simulink model "SimNL"  (R2016b)
settings: Solver=VariableStepAuto  StartTime=0.0  StopTime=10  FixedStep=SampleTime  RelTol=1e-3
undefined symbols (not defined in the file): AC, Sim
libraries: Surf_Lib x7, OpenFlightUtilLib x5, SimCoreLib x2, EnvLib x1
settings Model: Creator=Paul Freeman  LastModifiedBy=rega0051
settings DataIOCC: SaveState=on
settings OptimizationCC: ExpressionDepthLimit=2147483647  LifeSpan=inf
settings DebuggingCC: SignalInfNanChecking=warning  SaveWithParameterizedLinksMsg=none  UnderspecifiedInitializationDetection=Classic  MergeDetectMultiDrivingBlocksExec=none  CheckMatrixSingularityMsg=warning  UnnecessaryDatatypeConvMsg=warning  FcnCallInpInsideContextMsg=warning  UnconnectedInputMsg=none  UnconnectedOutputMsg=none  UnconnectedLineMsg=none  SFcnCompatibilityMsg=warning  UniqueDataStoreMsg=warning  StateNameClashWarn=warning  SFUnexpectedBacktrackingDiag=warning  SFNoUnconditionalDefaultTransitionDiag=warning  SFExecutionAtInitializationDiag=none
settings HardwareCC: ProdBitPerPointer=32  ProdBitPerSizeT=32  ProdBitPerPtrDiffT=32  ProdLargestAtomicFloat=None  ProdWordSize=32  ProdHWDeviceType=Custom Processor->Custom
settings GRTTargetCC: TargetLangStandard=C89/C90 (ANSI)  GeneratePreprocessorConditionals=Disable all  CombineOutputUpdateFcns=off  GRTInterface=on
settings ConfigComp: CovMetricSettings=dw  CovHtmlReporting=on  CovSaveCumulativeToWorkspaceVar=on  CovSaveSingleToWorkspaceVar=on  CovExternalEMLEnable=off  CovSFcnEnable=off

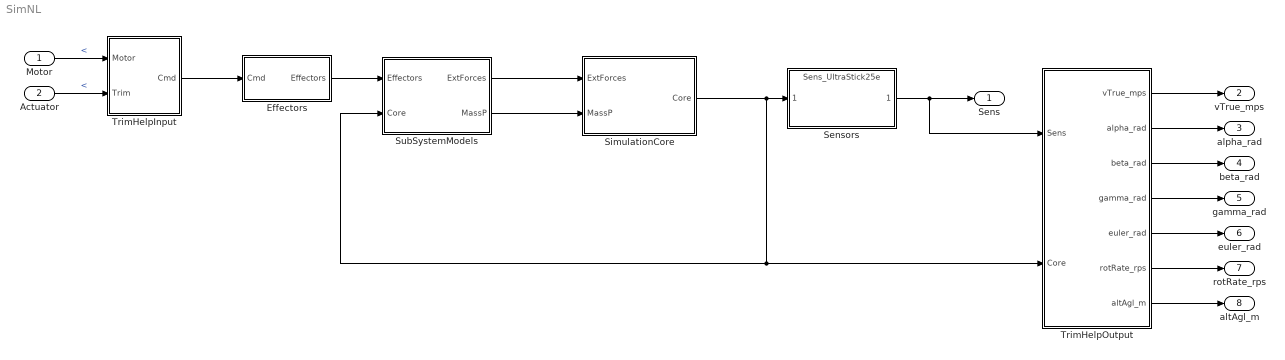
== system SimNL ==
  Motor : Inport
  Actuator : Inport  Port=2
  Effectors : Subsystem  TreatAsAtomicUnit=on
  Sensors : ModelReference  ModelNameDialog=Sens_UltraStick25e.slx  SimulationMode=Normal  ModelReferenceVersion=1.71
  SimulationCore : Subsystem
  SubSystemModels : Subsystem
  TrimHelpInput : Subsystem
  TrimHelpOutput : Subsystem
  Sens : Outport  OutDataTypeStr=Bus: BusSens
  vTrue_mps : Outport  Port=2
  alpha_rad : Outport  Port=3
  beta_rad : Outport  Port=4
  gamma_rad : Outport  Port=5
  euler_rad : Outport  Port=6
  rotRate_rps : Outport  Port=7
  altAgl_m : Outport  Port=8
  wires:
  SimulationCore/1(Core) -> TrimHelpOutput/2(Core), SubSystemModels/2(Core), Sensors/1
  Actuator/1 -> TrimHelpInput/2(Trim)  "<"
  Motor/1 -> TrimHelpInput/1(Motor)  "<"
  TrimHelpInput/1(Cmd) -> Effectors/1(Cmd)
  SubSystemModels/1(ExtForces) -> SimulationCore/1(ExtForces)
  SubSystemModels/2(MassP) -> SimulationCore/2(MassP)
  Sensors/1 -> TrimHelpOutput/1(Sens), Sens/1
  TrimHelpOutput/1(vTrue_mps) -> vTrue_mps/1
  TrimHelpOutput/2(alpha_rad) -> alpha_rad/1
  TrimHelpOutput/3(beta_rad) -> beta_rad/1
  TrimHelpOutput/4(gamma_rad) -> gamma_rad/1
  TrimHelpOutput/5(euler_rad) -> euler_rad/1
  TrimHelpOutput/6(rotRate_rps) -> rotRate_rps/1
  TrimHelpOutput/7(altAgl_m) -> altAgl_m/1
  Effectors/1(Effectors) -> SubSystemModels/1(Effectors)

== system SimNL/Effectors ==
  Cmd : Inport
  Bus Creator : BusCreator  Inputs=3  OutDataTypeStr=Bus: BusEff
      settings: AttributesFormatString=%<OutDataTypeStr>  InheritFromInputs=off
  ControlSurfaces : Subsystem
  MotorModels : Subsystem
  Effectors : Outport
  wires:
  ControlSurfaces/1(Act) -> Bus Creator/2
  MotorModels/1(Throttle) -> Bus Creator/1
  Cmd/1 -> MotorModels/1(Cmd), ControlSurfaces/1(Cmd)
  ControlSurfaces/2(Surf) -> Bus Creator/3
  Bus Creator/1 -> Effectors/1  "BusEff"

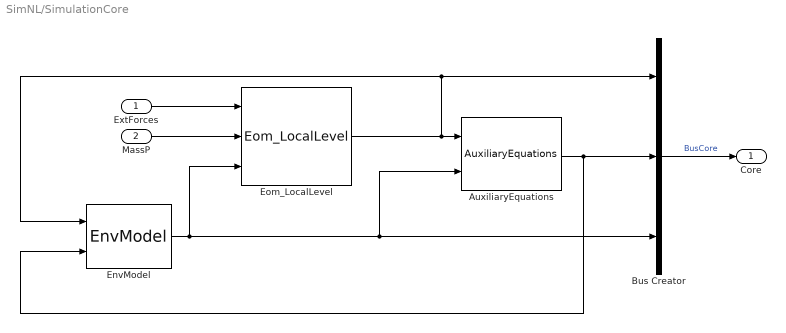
== system SimNL/SimulationCore ==
  ExtForces : Inport
  MassP : Inport  Port=2
  AuxiliaryEquations : SimCoreLib/AuxiliaryEquations
  Bus Creator : BusCreator  Inputs=3  OutDataTypeStr=Bus: BusCore
      settings: AttributesFormatString=%<OutDataTypeStr>
  EnvModel : EnvLib/EnvModel
  Eom_LocalLevel : SimCoreLib/Eom_LocalLevel  SystemSampleTime=-1
  Core : Outport
  wires:
  ExtForces/1 -> Eom_LocalLevel/1
  EnvModel/1 -> AuxiliaryEquations/2, Bus Creator/3, Eom_LocalLevel/3
  Bus Creator/1 -> Core/1  "BusCore"
  MassP/1 -> Eom_LocalLevel/2
  Eom_LocalLevel/1 -> EnvModel/1, Bus Creator/1, AuxiliaryEquations/1
  AuxiliaryEquations/1 -> EnvModel/2, Bus Creator/2

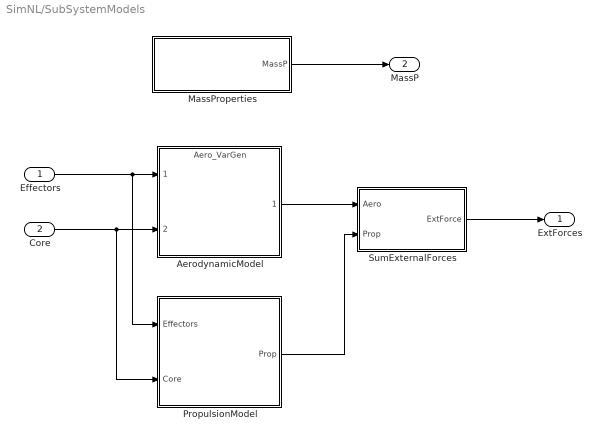
== system SimNL/SubSystemModels ==
  Effectors : Inport
  Core : Inport  Port=2
  AerodynamicModel : ModelReference  ModelNameDialog=Aero_VarGen  SimulationMode=Normal  Variant=on  ModelReferenceVersion=1.70
  MassProperties : Subsystem
  PropulsionModel : Subsystem
  SumExternalForces : Subsystem
  ExtForces : Outport
  MassP : Outport  Port=2
  wires:
  MassProperties/1(MassP) -> MassP/1
  AerodynamicModel/1 -> SumExternalForces/1(Aero)
  SumExternalForces/1(ExtForce) -> ExtForces/1
  PropulsionModel/1(Prop) -> SumExternalForces/2(Prop)
  Effectors/1 -> PropulsionModel/1(Effectors), AerodynamicModel/1
  Core/1 -> PropulsionModel/2(Core), AerodynamicModel/2

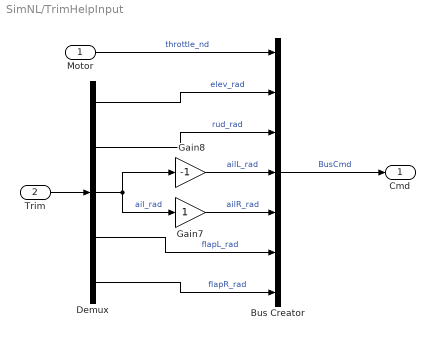
== system SimNL/TrimHelpInput ==
  Motor : Inport
  Trim : Inport  Port=2
  Bus Creator : BusCreator  Inputs=7  OutDataTypeStr=Bus: BusCmd
      settings: AttributesFormatString=%<OutDataTypeStr>
  Demux : Demux  Outputs=5
  Gain7 : Gain
  Gain8 : Gain  Gain=-1
  Cmd : Outport
  wires:
  Motor/1 -> Bus Creator/1  "throttle_nd"
  Demux/2 -> Bus Creator/3  "rud_rad"
  Demux/1 -> Bus Creator/2  "elev_rad"
  Trim/1 -> Demux/1
  Demux/5 -> Bus Creator/7  "flapR_rad"
  Demux/3 -> Gain7/1, Gain8/1  "ail_rad"
  Demux/4 -> Bus Creator/6  "flapL_rad"
  Gain7/1 -> Bus Creator/5  "ailR_rad"
  Gain8/1 -> Bus Creator/4  "ailL_rad"
  Bus Creator/1 -> Cmd/1  "BusCmd"

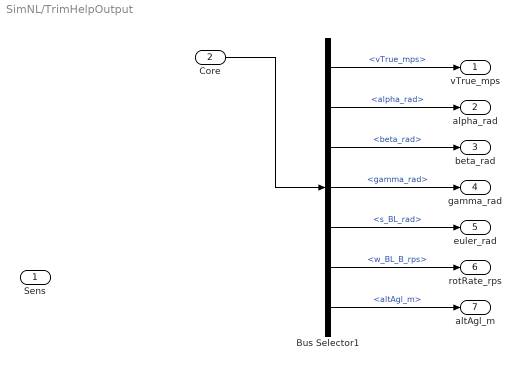
== system SimNL/TrimHelpOutput ==
  Sens : Inport
  Core : Inport  Port=2
  Bus Selector1 : BusSelector  OutputSignals=BusAux.BusFlow.vTrue_mps,BusAux.BusFlow.alpha_rad,BusAux.BusFlow.beta_rad,BusAux.BusNav.gamma_rad,BusEom.s_BL_rad,BusEom.w_BL_B_rps,BusAux.BusNav.altAgl_m
  vTrue_mps : Outport
  alpha_rad : Outport  Port=2
  beta_rad : Outport  Port=3
  gamma_rad : Outport  Port=4
  euler_rad : Outport  Port=5
  rotRate_rps : Outport  Port=6
  altAgl_m : Outport  Port=7
  wires:
  Core/1 -> Bus Selector1/1
  Bus Selector1/1 -> vTrue_mps/1  "<vTrue_mps>"
  Bus Selector1/3 -> beta_rad/1  "<beta_rad>"
  Bus Selector1/2 -> alpha_rad/1  "<alpha_rad>"
  Bus Selector1/4 -> gamma_rad/1  "<gamma_rad>"
  Bus Selector1/5 -> euler_rad/1  "<s_BL_rad>"
  Bus Selector1/6 -> rotRate_rps/1  "<w_BL_B_rps>"
  Bus Selector1/7 -> altAgl_m/1  "<altAgl_m>"

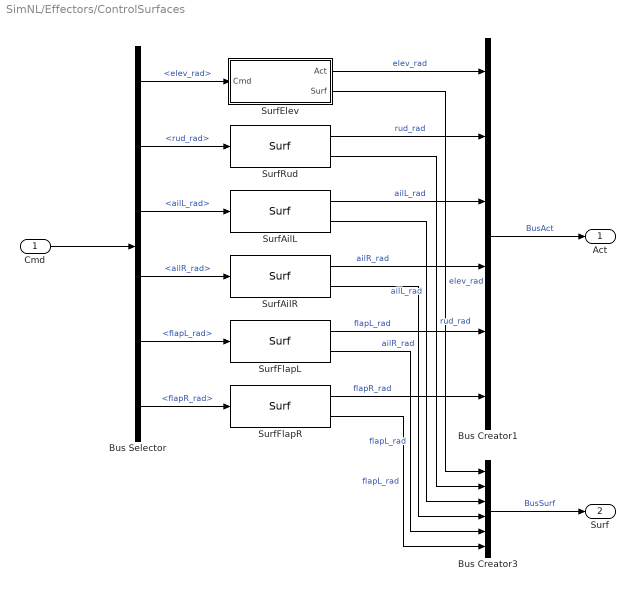
== system SimNL/Effectors/ControlSurfaces ==
  Cmd : Inport
  Bus Creator1 : BusCreator  Inputs=6  OutDataTypeStr=Bus: BusAct
      settings: AttributesFormatString=%<OutDataTypeStr>  InheritFromInputs=off
  Bus Creator3 : BusCreator  Inputs=6  OutDataTypeStr=Bus: BusSurf
      settings: AttributesFormatString=%<OutDataTypeStr>  InheritFromInputs=off
  Bus Selector : BusSelector  OutputSignals=elev_rad,rud_rad,ailL_rad,ailR_rad,flapL_rad,flapR_rad
  SurfAilL : Surf_Lib/Surf  surf=AC.Surf.ailL
  SurfAilR : Surf_Lib/Surf  surf=AC.Surf.ailR
  SurfElev : Subsystem  AncestorBlock=Surf_Lib/Surf  mask{surf=AC.Surf.elev}
      mask prompts: surf "Surface Structure:"
  SurfFlapL : Surf_Lib/Surf  surf=AC.Surf.flapL
  SurfFlapR : Surf_Lib/Surf  surf=AC.Surf.flapR
  SurfRud : Surf_Lib/Surf  surf=AC.Surf.rud
  Act : Outport
  Surf : Outport  Port=2
  wires:
  Bus Creator1/1 -> Act/1  "BusAct"
  Cmd/1 -> Bus Selector/1
  Bus Selector/1 -> SurfElev/1(Cmd)  "<elev_rad>"
  Bus Selector/2 -> SurfRud/1  "<rud_rad>"
  Bus Selector/3 -> SurfAilL/1  "<ailL_rad>"
  SurfAilL/1 -> Bus Creator1/3  "ailL_rad"
  Bus Selector/5 -> SurfFlapL/1  "<flapL_rad>"
  SurfFlapL/1 -> Bus Creator1/5  "flapL_rad"
  SurfAilR/1 -> Bus Creator1/4  "ailR_rad"
  SurfFlapR/1 -> Bus Creator1/6  "flapR_rad"
  Bus Selector/6 -> SurfFlapR/1  "<flapR_rad>"
  SurfRud/1 -> Bus Creator1/2  "rud_rad"
  Bus Selector/4 -> SurfAilR/1  "<ailR_rad>"
  SurfElev/2(Surf) -> Bus Creator3/1  "elev_rad"
  SurfRud/2 -> Bus Creator3/2  "rud_rad"
  SurfAilL/2 -> Bus Creator3/3  "ailL_rad"
  SurfAilR/2 -> Bus Creator3/4  "ailR_rad"
  SurfFlapL/2 -> Bus Creator3/5  "flapL_rad"
  SurfFlapR/2 -> Bus Creator3/6  "flapL_rad"
  Bus Creator3/1 -> Surf/1  "BusSurf"
  SurfElev/1(Act) -> Bus Creator1/1  "elev_rad"

== system SimNL/Effectors/MotorModels ==
  Cmd : Inport  OutDataTypeStr=double
  Bus Creator : BusCreator  Inputs=1
  Bus Selector1 : BusSelector  OutputSignals=throttle_nd
  Throttle : Outport
  wires:
  Cmd/1 -> Bus Selector1/1
  Bus Selector1/1 -> Bus Creator/1  "<throttle_nd>"
  Bus Creator/1 -> Throttle/1  "BusThrot"

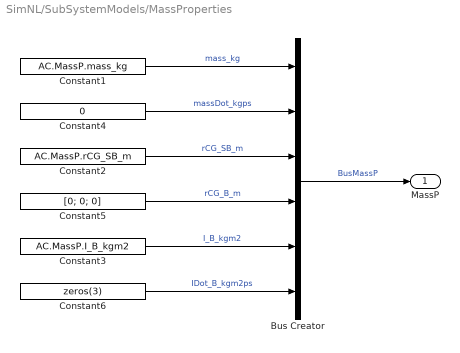
== system SimNL/SubSystemModels/MassProperties ==
  Bus Creator : BusCreator  Inputs=6  OutDataTypeStr=Bus: BusMassP
      settings: AttributesFormatString=%<OutDataTypeStr>
  Constant1 : Constant  Value=AC.MassP.mass_kg
      settings: AttributesFormatString=%<Value>
  Constant2 : Constant  Value=AC.MassP.rCG_SB_m
      settings: AttributesFormatString=%<Value>
  Constant3 : Constant  Value=AC.MassP.I_B_kgm2
      settings: AttributesFormatString=%<Value>
  Constant4 : Constant  Value=0
      settings: AttributesFormatString=%<Value>
  Constant5 : Constant  Value=[0; 0; 0]
      settings: AttributesFormatString=%<Value>
  Constant6 : Constant  Value=zeros(3)
      settings: AttributesFormatString=%<Value>
  MassP : Outport
  wires:
  Bus Creator/1 -> MassP/1  "BusMassP"
  Constant1/1 -> Bus Creator/1  "mass_kg"
  Constant2/1 -> Bus Creator/3  "rCG_SB_m"
  Constant3/1 -> Bus Creator/5  "I_B_kgm2"
  Constant4/1 -> Bus Creator/2  "massDot_kgps"
  Constant5/1 -> Bus Creator/4  "rCG_B_m"
  Constant6/1 -> Bus Creator/6  "IDot_B_kgm2ps"

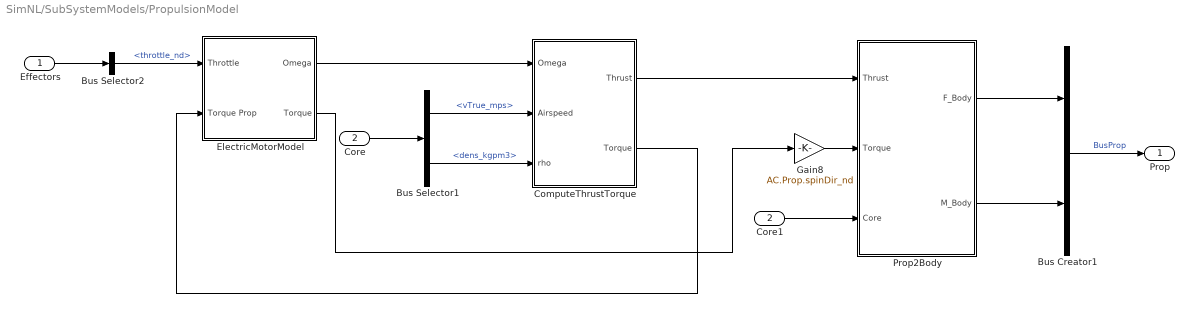
== system SimNL/SubSystemModels/PropulsionModel ==
  Effectors : Inport  OutDataTypeStr=double
  Core : Inport  Port=2
  Bus Selector1 : BusSelector  OutputSignals=BusAux.BusFlow.vTrue_mps,BusEnv.BusAtmos.dens_kgpm3
  Bus Selector2 : BusSelector  OutputSignals=BusThrot.throttle_nd
  Bus Creator1 : BusCreator  Inputs=2  OutDataTypeStr=Bus: BusProp
      settings: AttributesFormatString=%<OutDataTypeStr>
  ComputeThrustTorque : Subsystem
  Core1 : InportShadow  Port=2
  ElectricMotorModel : Subsystem  mask{motor=AC.Motor}
      mask prompts: motor "Motor Parameter Structure:"
  Gain8 : Gain  Gain=AC.Prop.spinDir_nd  SaturateOnIntegerOverflow=on  OutDataTypeStr=Inherit: Same as input  ParamDataTypeStr=Inherit: Same as input
      settings: AttributesFormatString=%<Gain>
  Prop2Body : Subsystem
  Prop : Outport
  wires:
  Core/1 -> Bus Selector1/1
  Prop2Body/2(M_Body) -> Bus Creator1/2
  ComputeThrustTorque/1(Thrust) -> Prop2Body/1(Thrust)
  Bus Selector1/1 -> ComputeThrustTorque/2(Airspeed)  "<vTrue_mps>"
  Prop2Body/1(F_Body) -> Bus Creator1/1
  Core1/1 -> Prop2Body/3(Core)
  Bus Creator1/1 -> Prop/1  "BusProp"
  Bus Selector1/2 -> ComputeThrustTorque/3(rho)  "<dens_kgpm3>"
  ElectricMotorModel/2(Torque) -> Gain8/1
  ComputeThrustTorque/2(Torque) -> ElectricMotorModel/2(Torque Prop)
  Effectors/1 -> Bus Selector2/1
  Gain8/1 -> Prop2Body/2(Torque)
  Bus Selector2/1 -> ElectricMotorModel/1(Throttle)  "<throttle_nd>"
  ElectricMotorModel/1(Omega) -> ComputeThrustTorque/1(Omega)

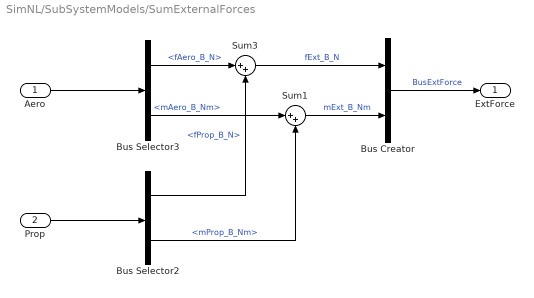
== system SimNL/SubSystemModels/SumExternalForces ==
  Aero : Inport
  Prop : Inport  Port=2
  Bus Selector2 : BusSelector  OutputSignals=fProp_B_N,mProp_B_Nm
  Bus Selector3 : BusSelector  OutputSignals=fAero_B_N,mAero_B_Nm
  Bus Creator : BusCreator  Inputs=2  OutDataTypeStr=Bus: BusExtForce
      settings: AttributesFormatString=%<OutDataTypeStr>
  Sum1 : Sum  Inputs=|++  SaturateOnIntegerOverflow=on
  Sum3 : Sum  Inputs=|++  SaturateOnIntegerOverflow=on
  ExtForce : Outport
  wires:
  Sum1/1 -> Bus Creator/2  "mExt_B_Nm"
  Sum3/1 -> Bus Creator/1  "fExt_B_N"
  Bus Creator/1 -> ExtForce/1  "BusExtForce"
  Prop/1 -> Bus Selector2/1
  Bus Selector2/1 -> Sum3/2  "<fProp_B_N>"
  Bus Selector2/2 -> Sum1/2  "<mProp_B_Nm>"
  Aero/1 -> Bus Selector3/1
  Bus Selector3/1 -> Sum3/1  "<fAero_B_N>"
  Bus Selector3/2 -> Sum1/1  "<mAero_B_Nm>"

== system SimNL/Effectors/ControlSurfaces/SurfElev ==
  Cmd : Inport
  LinkageModel : Subsystem  BlockChoice=LinkageModel_Lin
      settings: AttributesFormatString=%<BlockChoice>  TemplateBlock=Surf_Lib/LinkageModel  MemberBlocks=LinkageModel_Lin,LinkageModel_NL,LinkageModel_Pass
  ServoModel : Subsystem  BlockChoice=ServoModel_2ndLin
      settings: AttributesFormatString=%<BlockChoice>  TemplateBlock=Surf_Lib/ServoModel  MemberBlocks=ServoModel_1stLin,ServoModel_1stNL,ServoModel_2ndLin,ServoModel_2ndNL
  Act : Outport
  Surf : Outport  Port=2
  wires:
  LinkageModel/1(Surf) -> Surf/1
  ServoModel/1(Act) -> Act/1, LinkageModel/1(Act)
  Cmd/1 -> ServoModel/1(Cmd)

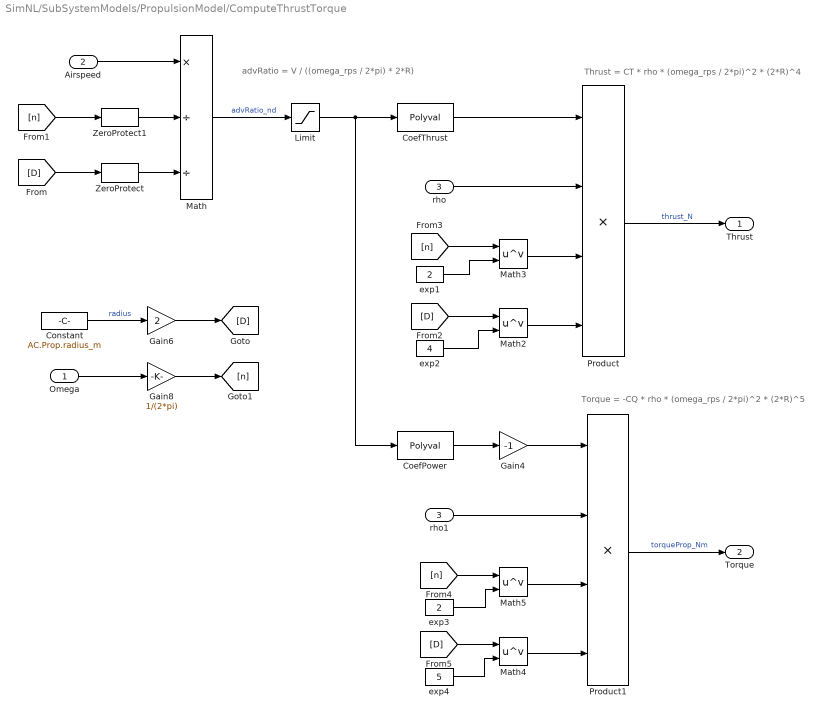
== system SimNL/SubSystemModels/PropulsionModel/ComputeThrustTorque ==
  note: advRatio = V / ((omega_rps / 2*pi) * 2*R)
  note: Thrust = CT * rho * (omega_rps / 2*pi)^2 * (2*R)^4
  note: Torque = -CQ * rho * (omega_rps / 2*pi)^2 * (2*R)^5
  Omega : Inport  OutDataTypeStr=double
  Airspeed : Inport  Port=2  OutDataTypeStr=double
  rho : Inport  Port=3  OutDataTypeStr=double
  CoefPower : Polyval  Coefs=AC.Prop.CQ
      settings: AttributesFormatString=%<Coefs>
  CoefThrust : Polyval  Coefs=AC.Prop.CT
      settings: AttributesFormatString=%<Coefs>
  Constant : Constant  Value=AC.Prop.radius_m
      settings: AttributesFormatString=%<Value>
  Gain4 : Gain  Gain=-1  SaturateOnIntegerOverflow=on  OutDataTypeStr=Inherit: Same as input  ParamDataTypeStr=Inherit: Same as input
  Gain6 : Gain  Gain=2  SaturateOnIntegerOverflow=on  OutDataTypeStr=Inherit: Same as input  ParamDataTypeStr=Inherit: Same as input
  Gain8 : Gain  Gain=1/(2*pi)  SaturateOnIntegerOverflow=on  OutDataTypeStr=Inherit: Same as input  ParamDataTypeStr=Inherit: Same as input
      settings: AttributesFormatString=%<Gain>
  Limit : Saturate  UpperLimit=0.7  LowerLimit=0
  Math : Product  Inputs=*//  SaturateOnIntegerOverflow=on  InputSameDT=on  OutDataTypeStr=Inherit: Same as first input
  Math{2..5} (4 alike) : Math  Operator=pow  SaturateOnIntegerOverflow=on
  Product : Product  Inputs=4  SaturateOnIntegerOverflow=on  InputSameDT=on  OutDataTypeStr=Inherit: Same as first input
  Product1 : Product  Inputs=4  SaturateOnIntegerOverflow=on  InputSameDT=on  OutDataTypeStr=Inherit: Same as first input
  ZeroProtect : OpenFlightUtilLib/Math/ZeroProtect  epsilon=eps
  ZeroProtect1 : OpenFlightUtilLib/Math/ZeroProtect  epsilon=eps
  exp1 : Constant  Value=2
  exp2 : Constant  Value=4
  exp3 : Constant  Value=2
  exp4 : Constant  Value=5
  rho1 : InportShadow  Port=3  OutDataTypeStr=double
  Thrust : Outport
  Torque : Outport  Port=2
  wires:
  CoefPower/1 -> Gain4/1
  CoefThrust/1 -> Product/1
  Product/1 -> Thrust/1  "thrust_N"
  Math2/1 -> Product/4
  exp2/1 -> Math2/2
  Math3/1 -> Product/3
  Math/1 -> Limit/1  "advRatio_nd"
  rho/1 -> Product/2
  Airspeed/1 -> Math/1
  Product1/1 -> Torque/1  "torqueProp_Nm"
  Limit/1 -> CoefThrust/1, CoefPower/1
  [n] -> Math3/1
  [D] -> Math2/1
  exp1/1 -> Math3/2
  Math4/1 -> Product1/4
  exp4/1 -> Math4/2
  Math5/1 -> Product1/3
  [n] -> Math5/1
  [D] -> Math4/1
  exp3/1 -> Math5/2
  rho1/1 -> Product1/2
  Gain4/1 -> Product1/1
  Gain6/1 -> [D]
  Constant/1 -> Gain6/1  "radius"
  Omega/1 -> Gain8/1
  Gain8/1 -> [n]
  [n] -> ZeroProtect1/1
  [D] -> ZeroProtect/1
  ZeroProtect/1 -> Math/3
  ZeroProtect1/1 -> Math/2

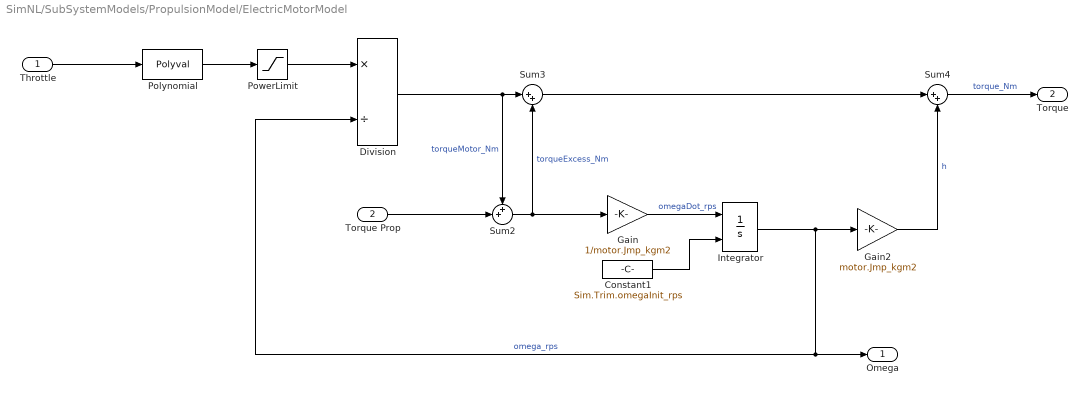
== system SimNL/SubSystemModels/PropulsionModel/ElectricMotorModel ==
  Throttle : Inport
  Torque Prop : Inport  Port=2
  Constant1 : Constant  Value=Sim.Trim.omegaInit_rps
      settings: AttributesFormatString=%<Value>
  Division : Product  Inputs=*/  SaturateOnIntegerOverflow=on  InputSameDT=on  OutDataTypeStr=Inherit: Same as first input
  Gain : Gain  Gain=1/motor.Jmp_kgm2
      settings: AttributesFormatString=%<Gain>
  Gain2 : Gain  Gain=motor.Jmp_kgm2  SaturateOnIntegerOverflow=on  OutDataTypeStr=Inherit: Same as input  ParamDataTypeStr=Inherit: Same as input
      settings: AttributesFormatString=%<Gain>
  Integrator : Integrator  InitialConditionSource=external  LimitOutput=on  UpperSaturationLimit=motor.omegaLimPos_rps  LowerSaturationLimit=motor.omegaLimNeg_rps  ContinuousStateAttributes='omegaState_rps'
      settings: AttributesFormatString=State: %<ContinuousStateAttributes>
  Polynomial : Polyval  Coefs=motor.power_w
  PowerLimit : Saturate  UpperLimit=motor.powerLimPos_w  LowerLimit=motor.powerLimNeg_w
  Sum2 : Sum  Inputs=++|  SaturateOnIntegerOverflow=on
  Sum3 : Sum  Inputs=|++  SaturateOnIntegerOverflow=on
  Sum4 : Sum  Inputs=|++  SaturateOnIntegerOverflow=on
  Omega : Outport
  Torque : Outport  Port=2
  wires:
  Throttle/1 -> Polynomial/1
  Sum3/1 -> Sum4/1
  Constant1/1 -> Integrator/2
  Gain/1 -> Integrator/1  "omegaDot_rps"
  Sum2/1 -> Sum3/2, Gain/1  "torqueExcess_Nm"
  Integrator/1 -> Omega/1, Division/2, Gain2/1  "omega_rps"
  Gain2/1 -> Sum4/2  "h"
  Sum4/1 -> Torque/1  "torque_Nm"
  PowerLimit/1 -> Division/1
  Polynomial/1 -> PowerLimit/1
  Division/1 -> Sum2/1, Sum3/1  "torqueMotor_Nm"
  Torque Prop/1 -> Sum2/2

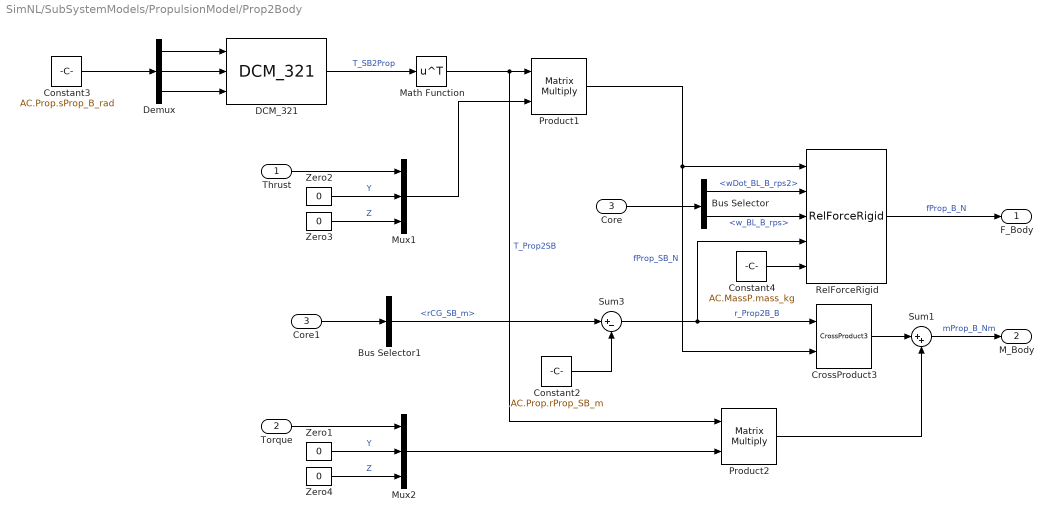
== system SimNL/SubSystemModels/PropulsionModel/Prop2Body ==
  Thrust : Inport
  Torque : Inport  Port=2
  Core : Inport  Port=3
  Bus Selector : BusSelector  OutputSignals=BusEom.wDot_BL_B_rps2,BusEom.w_BL_B_rps
  Bus Selector1 : BusSelector  OutputSignals=BusEom.rCG_SB_m
  Constant2 : Constant  Value=AC.Prop.rProp_SB_m
      settings: AttributesFormatString=%<Value>
  Constant3 : Constant  Value=AC.Prop.sProp_B_rad
      settings: AttributesFormatString=%<Value>
  Constant4 : Constant  Value=AC.MassP.mass_kg
      settings: AttributesFormatString=%<Value>
  Core1 : InportShadow  Port=3
  CrossProduct3 : OpenFlightUtilLib/Math/CrossProduct3
  DCM_321 : OpenFlightUtilLib/Transformations/DCM_321
  Demux : Demux  Outputs=3
  Math Function : Math  Operator=transpose  SaturateOnIntegerOverflow=on
  Mux1 : Mux  Inputs=3
  Mux2 : Mux  Inputs=3
  Product1 : Product  Multiplication=Matrix(*)  RndMeth=Zero
  Product2 : Product  Multiplication=Matrix(*)  RndMeth=Zero
  RelForceRigid : OpenFlightUtilLib/Kinematics and Dynamics/RelForceRigid
  Sum1 : Sum  Inputs=|++  SaturateOnIntegerOverflow=on
  Sum3 : Sum  Inputs=|+-  SaturateOnIntegerOverflow=on
  Zero{1..4} (4 alike) : Constant  Value=0
  F_Body : Outport
  M_Body : Outport  Port=2
  wires:
  Bus Selector1/1 -> Sum3/1  "<rCG_SB_m>"
  Constant2/1 -> Sum3/2
  Bus Selector/1 -> RelForceRigid/2  "<wDot_BL_B_rps2>"
  Bus Selector/2 -> RelForceRigid/3  "<w_BL_B_rps>"
  Thrust/1 -> Mux1/1
  Math Function/1 -> Product2/1, Product1/1  "T_Prop2SB"
  Product1/1 -> RelForceRigid/1, CrossProduct3/2  "fProp_SB_N"
  Sum3/1 -> CrossProduct3/1, RelForceRigid/4  "r_Prop2B_B"
  Core/1 -> Bus Selector/1
  RelForceRigid/1 -> F_Body/1  "fProp_B_N"
  CrossProduct3/1 -> Sum1/1
  Sum1/1 -> M_Body/1  "mProp_B_Nm"
  Constant3/1 -> Demux/1
  Demux/3 -> DCM_321/3
  Demux/1 -> DCM_321/1
  Demux/2 -> DCM_321/2
  DCM_321/1 -> Math Function/1  "T_SB2Prop"
  Product2/1 -> Sum1/2
  Constant4/1 -> RelForceRigid/5
  Zero3/1 -> Mux1/3  "Z"
  Zero2/1 -> Mux1/2  "Y"
  Mux1/1 -> Product1/2
  Zero4/1 -> Mux2/3  "Z"
  Zero1/1 -> Mux2/2  "Y"
  Torque/1 -> Mux2/1
  Mux2/1 -> Product2/2
  Core1/1 -> Bus Selector1/1

== system SimNL/Effectors/ControlSurfaces/SurfElev/LinkageModel ==
  Act : Inport
  LinkageModel_Lin : Surf_Lib/LinkageModel_Lin  VariantControl=VarLink_Lin
  Surf : Outport
  wires:
  Act/1 -> LinkageModel_Lin/1
  LinkageModel_Lin/1 -> Surf/1

== system SimNL/Effectors/ControlSurfaces/SurfElev/ServoModel ==
  Cmd : Inport
  ServoModel_2ndLin : Surf_Lib/ServoModel_2ndLin  VariantControl=VarServo_NL1
  Act : Outport
  wires:
  Cmd/1 -> ServoModel_2ndLin/1
  ServoModel_2ndLin/1 -> Act/1
